simulink model "Parent"  (R2023a)
settings: Solver=VariableStepAuto  StartTime=0.0  StopTime=10.0  RelTol=1e-3
libraries: androidcommunicationlib x4, androidaudiovideolib x2, androiduilib x2
settings Model: Creator=DELL  LastModifiedBy=abhimanyuyadav

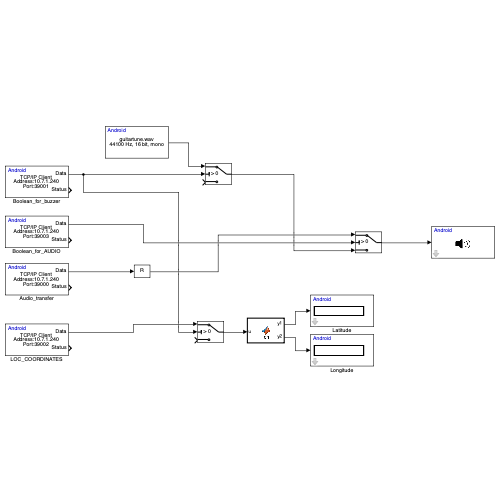
[thumbnail: Simulink's stored preview of the top-level diagram]
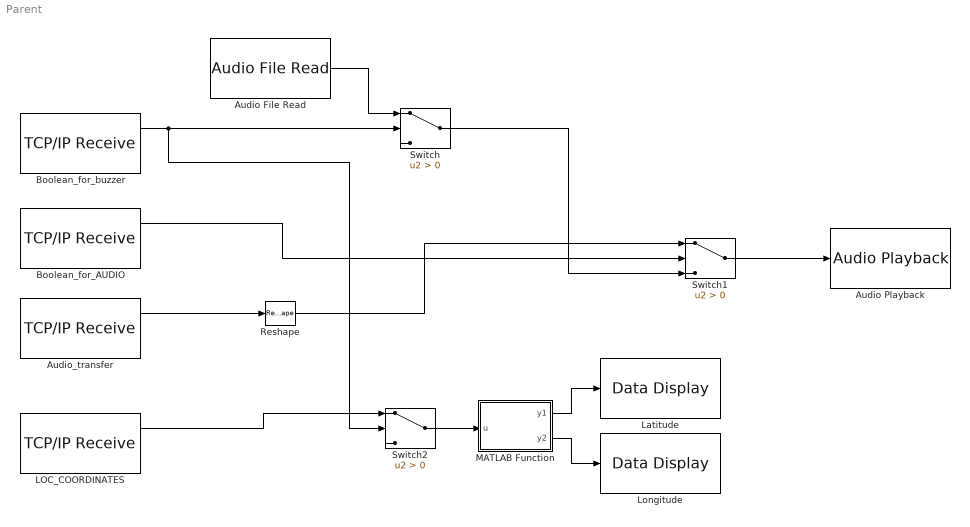
== system Parent ==
  Audio File Read : androidaudiovideolib/Audio File Read  FileName=C:\Users\DELL\Downloads\emergency-alarm-with-reverb-29431.mp3  FrameSize=4410
  Audio Playback : androidaudiovideolib/Audio Playback  SampleFreq=44100  AudioSamplingFreq=44100  SampleTime=0.1  DeviceStr=0  QueueDuration=0  BlockPlatform=Android
  Audio_transfer : androidcommunicationlib/TCP//IP Receive  Mode_=Client  LocalServerPort_=25000  RemoteAddr_=10.7.1.240  RemoteServerPort_=39000  DataType_=int16  DataSize_=8820  SampleTime_=0.1  ClientPortBindingSelection_=off  ClientPortToBind_=35000  BlockingMode_=off  BlockTimeout_=0.1
  Boolean_for_AUDIO : androidcommunicationlib/TCP//IP Receive  Mode_=Client  LocalServerPort_=25000  RemoteAddr_=10.7.1.240  RemoteServerPort_=39003  DataType_=boolean  DataSize_=1  SampleTime_=0.1  ClientPortBindingSelection_=off  ClientPortToBind_=35000  BlockingMode_=off  BlockTimeout_=0.1
  Boolean_for_buzzer : androidcommunicationlib/TCP//IP Receive  Mode_=Client  LocalServerPort_=25000  RemoteAddr_=10.7.1.240  RemoteServerPort_=39001  DataType_=boolean  DataSize_=1  SampleTime_=0.1  ClientPortBindingSelection_=off  ClientPortToBind_=35000  BlockingMode_=off  BlockTimeout_=0.1
  LOC_COORDINATES : androidcommunicationlib/TCP//IP Receive  Mode_=Client  LocalServerPort_=25000  RemoteAddr_=10.7.1.240  RemoteServerPort_=39002  DataType_=double  DataSize_=2  SampleTime_=0.1  ClientPortBindingSelection_=off  ClientPortToBind_=35000  BlockingMode_=off  BlockTimeout_=0.1
  Latitude : androiduilib/Data Display  Format=Float  Precision=6  SimulateUsing=Code generation  blockPlatform=Android
  Longitude : androiduilib/Data Display  Format=Float  Precision=6  SimulateUsing=Code generation  blockPlatform=Android
  MATLAB Function : MATLAB Function  TreatAsAtomicUnit=on
  Reshape : Reshape  OutputDimensionality=Customize  OutputDimensions=[4410,2]
  Switch : Switch  Criteria=u2 > Threshold  SaturateOnIntegerOverflow=off  InputSameDT=off
  Switch1 : Switch  Criteria=u2 > Threshold  SaturateOnIntegerOverflow=off  InputSameDT=off
  Switch2 : Switch  Criteria=u2 > Threshold  SaturateOnIntegerOverflow=off  InputSameDT=off
  wires:
  Audio_transfer/1 -> Reshape/1
  Switch1/1 -> Audio Playback/1
  Boolean_for_buzzer/1 -> Switch2/2, Switch/2
  Audio File Read/1 -> Switch/1
  Switch/1 -> Switch1/3
  Switch2/1 -> MATLAB Function/1(u)
  MATLAB Function/1(y1) -> Latitude/1
  MATLAB Function/2(y2) -> Longitude/1
  Boolean_for_AUDIO/1 -> Switch1/2
  Reshape/1 -> Switch1/1
  LOC_COORDINATES/1 -> Switch2/1

== matlab function Parent/MATLAB Function ==
  data: u input; y1 output; y2 output
function [y1,y2] = fcn(u)
y1=u(1);
y2=u(2);
y = u;
